simulink subsystem "Reference_step"  (R2024b)
settings: Solver=VariableStepAuto  StartTime=0.0  StopTime=10.0  RelTol=1e-3
undefined symbols (not defined in the file): ref_pos_length, step_delay_time, step_interval_time
settings Model: Creator=tshintai  LastModifiedBy=tshintai
settings OptimizationCC: ReuseModelBlockBuffer=off
settings ModelReferenceCC: EnableRefExpFcnMdlSchedulingChecks=on
settings RTWCC: GPUComputeCapability=3.5

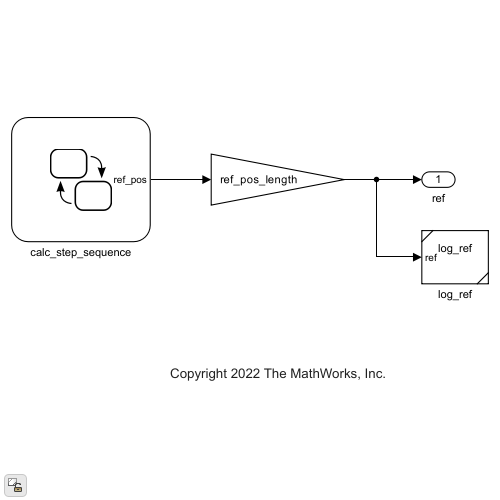
[thumbnail: Simulink's stored preview of the top-level diagram]
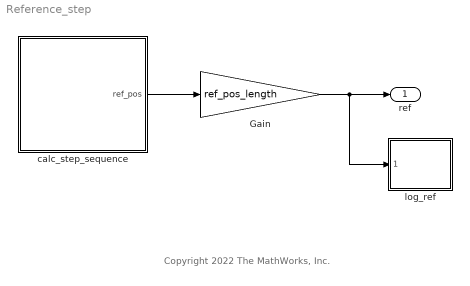
== system Reference_step ==
  note: Copyright 2022 The MathWorks, Inc.
  Gain : Gain  Gain=ref_pos_length
  calc_step_sequence : Stateflow chart  TreatAsAtomicUnit=on
  log_ref : Subsystem  ReferencedSubsystem=log_ref
  ref : Outport
  wires:
  calc_step_sequence/1(ref_pos) -> Gain/1
  Gain/1 -> log_ref/1, ref/1

== stateflow chart Reference_step/calc_step_sequence ==
  state INITIAL_WAIT
    entry:
    ref_pos = [0; 0];
  state MODE_INIT
    entry:
    ref_pos = [1; 0];
  state MODE_PP
    entry:
    ref_pos = [1; 1];
  state MODE_NP
    entry:
    ref_pos = [-1; 1];
  state MODE_PN
    entry:
    ref_pos = [1; -1];
  state MODE_NN
    entry:
    ref_pos = [-1; -1];
  (default) -> INITIAL_WAIT
  INITIAL_WAIT -> MODE_INIT : [
      | after(step_delay_time, sec)
      | ]
  MODE_INIT -> MODE_PP : [
      | after(step_interval_time, sec)
      | ]
  MODE_PP -> MODE_NP : [
      | after(step_interval_time, sec)
      | ]
  MODE_PN -> MODE_PP : [
      | after(step_interval_time, sec)
      | ]
  MODE_NP -> MODE_NN : [
      | after(step_interval_time, sec)
      | ]
  MODE_NN -> MODE_PN : [
      | after(step_interval_time, sec)
      | ]
  data: ref_pos output; step_delay_time parameter; step_interval_time parameter
